simulink model "UPSControl"  (R2025b)
settings: Solver=VariableStepAuto  StartTime=0.0  StopTime=10  FixedStep=Ts  RelTol=1e-3
PostLoadFcn:
  | DataCenterParam;
values from neighbouring files (symbols this model uses):
  generator = struct    [GeneratorParam.m]
  lineInductance = 1e-6    (= 1e-06)    [DataCenterParam.m]    (also in GridParam.m)
  lineResistance = 1e-3    (= 0.001)    [DataCenterParam.m]    (also in GridParam.m)
  loadPower = 5e6    (= 5000000)    [DataCenterParam.m]    (also in LVRT.m; RedundancyAnalysis.m = 10000000)
  machine = struct    [GeneratorParam.m]
  powerTau = 0.005    [DataCenterParam.m]
  Ts = 5e-5    (= 5e-05)    [DataCenterParam.m]    (also in GeneratorParam.m)
  utilizationFactor = 0.45    [DataCenterParam.m]    (also in RedundancyAnalysis.m)
undefined symbols (not defined in the file or in its folder): breaker, ctLimitDelayTime, DiscIntNeverNeededParam, ee_sli_rtmsupport, gcbh, grid, rack, ups
libraries: nesl_utility x96, fl_lib x96, eeGeneralControl x84, ee_lib x80, simulink x68, eeTransforms x30, nesl_utility_internal x16, eeSinusoidalMeasurementV2 x13, slpidlib x12, simulink_extras x12, datacenter_lib x5, batteryecm_lib x4
(part 2 of 13)

== system UPSControl/ Back up Generator/Generator Set/Detailed ==
  PRef : Inport
  AVR and Exciter : Subsystem
  "Governor and Prime Mover " : Subsystem  mask(Governor and Prime Mover){pu_speed_reference=pu_speed_reference, droop_percentage=droop_percentage, pu_load_reference_setpoint=pu_load_reference_setpoint, T_G=T_G, T_CH=T_CH, base_torque=base_torque, pu_torque0=pu_torque0}
      mask prompts: pu_speed_reference "Speed reference, (pu)"; droop_percentage "Percentage droop, (%)"; pu_load_reference_setpoint "Load reference setpoint, (pu)"; T_G "Time constant of governor, (s)"; T_CH "Time constant of main inlet volumes and steam chest, (s)"; base_torque "Base torque, (N*m)"; pu_torque0 "Initial torque, (pu)"
      mask help:
      | Implements a synchronous machine governor and prime mover. The prime mover is a non-reheat steam turbine.
      |
      | The input to the block is a per-unit synchronous machine measurement vector.
      |
      | R and C are mechanical rotational ports.
  Inertia : ee_lib/Electromechanical/Mechanical/Machine Inertia  SRated=genRating*1000 V*A  FRated=frequency Hz  nPolePairs=polePairs  inertia_option=2  J=0.5754*200 kg*m^2  H=3.525*4 s*W/V/A  damper_option=2  D=39.0509 N*m/(rad/s)  pu_D=0.01  initialization_option=2  fMechanical0=30 Hz  fElectrical0=frequency Hz
      settings: InternalSimscapePortConfiguration="{\"Bottom\":[],\"Left\":[{\"id\":\"R\",\"label\":\"R\",\"type\":\"foundation.mechanical.rotational.rotational\"}],\"Right\":[],\"Top\":[]}"
  Machine : ee_lib/Electromechanical/Synchronous/Synchronous Machine Round Rotor  port_option=ee.enum.threePhasePort.composite  SRated=genRating*1000 A*V  VRated=Vac V  FRated=frequency Hz  nPolePairs=polePairs  param_option=ee.enum.sm.parameterization.standard  fieldCircuitParameterization_option=ee.enum.sm.fieldparameterization.voltage  baseEfd=200 V  baseIfd=1e-3%machine.fieldCurrent A  zero_sequence=ee.enum.park.zerosequence.exclude  axes_param=ee.enum.rotorangle.daxis  Ladu=1.66  Laqu=1.61  L0=0.15  Ll=0.05  Ra=machine.Ra  Lfd=0.165  Rfd=0.0006  L1d=0.1713  R1d=0.0284  L1q=0.7252  R1q=0.00619  L2q=0.125  R2q=0.02368  Xl=machine.Xl  Xd=machine.Xd  Xq=machine.Xq  X0=0.06  Xdd=machine.XdTransient  Xqd=machine.XqTransient  Xddd=machine.XdSubTransient  Xqdd=machine.XqSubTransient  d_option=ee.enum.circuit.open  Td0d=machine.tauDAxisTransient s  Tdd=0.03 s  Td0dd=machine.tauDAxisSubTransient s  Tddd=0.008 s  q_option=ee.enum.circuit.open  Tq0d=machine.tauQAxisTransient s  Tqd=0.03 s  Tq0dd=machine.tauQAxisSubTransient s  Tqdd=0.008 s  saturation_option=ee.enum.saturation.exclude  saturation_ifd=[0, .48, .76, 1.38, 1.79]  saturation_Vag=[0, .8, 1.08, 1.31, 1.4]  initialization_option=ee.enum.sm.initialization.electrical  source_type=ee.enum.sm.load_flow_source_type.Swing  Vmag0=machine.voltage V  Vang0=0 deg  Pt0=0 A*V  Qt0=0 A*V  minimum_pu=0.95  phase_search_range=[-inf, inf] deg  gmin=1e-6 S  connection_option=ee.enum.Connection.wye  num_q_dampers=2  rotor_offset=-pi / 2 rad  pu_psid_specify=off  pu_psid_priority=None  pu_psid=0  pu_psid_nominal_specify=off  pu_psid_nominal_value=1  pu_psid_nominal_unit=1  pu_psiq_specify=off  pu_psiq_priority=None  pu_psiq=0  pu_psiq_nominal_specify=off  pu_psiq_nominal_value=1  pu_psiq_nominal_unit=1  pu_psifd_specify=off  pu_psifd_priority=None  pu_psifd=0  pu_psifd_nominal_specify=off  pu_psifd_nominal_value=1  pu_psifd_nominal_unit=1  pu_psi1d_specify=off  pu_psi1d_priority=None  pu_psi1d=0  pu_psi1d_nominal_specify=off  pu_psi1d_nominal_value=1  pu_psi1d_nominal_unit=1  pu_psi1q_specify=off  pu_psi1q_priority=None  pu_psi1q=0  pu_psi1q_nominal_specify=off  pu_psi1q_nominal_value=1  pu_psi1q_nominal_unit=1  pu_psi2q_specify=off  pu_psi2q_priority=None  pu_psi2q=0  pu_psi2q_nominal_specify=off  pu_psi2q_nominal_value=1  pu_psi2q_nominal_unit=1  angular_position_diff_specify=off  angular_position_diff_priority=None  angular_position_diff=180 deg  angular_position_diff_nominal_specify=off  angular_position_diff_nominal_value=1  angular_position_diff_nominal_unit=deg  Tmeas=298.15 K  alpha=3.93e-3 1/K  stator_thermal_mass=100 J/K  rotor_thermal_mass=200 J/K  temperatureA_specify=off  temperatureA_priority=High  temperatureA=25 degC  temperatureA_nominal_specify=off  temperatureA_nominal_value=1  temperatureA_nominal_unit=degC  temperatureB_specify=off  temperatureB_priority=High  temperatureB=25 degC  temperatureB_nominal_specify=off  temperatureB_nominal_value=1  temperatureB_nominal_unit=degC  temperatureC_specify=off  temperatureC_priority=High  temperatureC=25 degC  temperatureC_nominal_specify=off  temperatureC_nominal_value=1  temperatureC_nominal_unit=degC  temperatureR_specify=off  temperatureR_priority=High  temperatureR=25 degC  temperatureR_nominal_specify=off  temperatureR_nominal_value=1  temperatureR_nominal_unit=degC
      settings: InternalSimscapePortConfiguration="{\"Bottom\":[],\"Left\":[{\"id\":\"fd_p\",\"label\":\"fd+\",\"type\":\"foundation.electrical.electrical\"},{\"id\":\"fd_n\",\"label\":\"fd-\",\"type\":\"foundation.electrical.electrical\"},{\"id\":\"R\",\"label\":\"R\",\"type\":\"foundation.mechanical.rotational.rotational\"},{\"id\":\"C\",\"label\":\"C\",\"type\":\"foundation.mechanical.rotational.rotational\"}],\"Right\":[{\"id\":\"pu_output\",\"label\":\"pu\",\"type\":\"output\"},{\"id\":\"N\",\"label\":\"~\",\"type\":\"foundation.electrical.three_phase\"}],\"Top\":[]}"
  Measurements : Subsystem
  ~ : PMIOPort  Side=Right
  Bus Element Out : Outport  PortName=Meas  Element=activePower
  BusElementOut : Outport  PortName=Meas  Element=reactivePower
  BusElementOut1 : Outport  PortName=Meas  Element=voltage
  BusElementOut2 : Outport  PortName=Meas  Element=current
  wires:
  Measurements/4(I) -> BusElementOut2/1
  Measurements/3(V) -> BusElementOut1/1
  Measurements/1(P) -> Bus Element Out/1
  Measurements/2(Q) -> BusElementOut/1
  PRef/1 -> "Governor and Prime Mover "/1(PRef)
  connections:
  ~/RConn1 -- Measurements/RConn1
  Measurements/LConn1 -- Machine/RConn2
  Machine/LConn1 -- AVR and Exciter/RConn1
  Machine/LConn4 -- "Governor and Prime Mover "/RConn2
  "Governor and Prime Mover "/RConn1 -- Machine/LConn3 -- Inertia/LConn1
  "Governor and Prime Mover "/LConn1 -- Machine/RConn1 -- AVR and Exciter/LConn1
  Machine/LConn2 -- AVR and Exciter/RConn2

== system UPSControl/ Back up Generator/Generator Set/Simplified ==
  PRef : Inport
  Electrical Reference : fl_lib/Electrical/Electrical Elements/Electrical Reference
  Exciter : Subsystem
  Machine : ee_lib/Electromechanical/Synchronous/Synchronous Machine Round Rotor  port_option=ee.enum.threePhasePort.composite  SRated=genRating kW  VRated=Vac V  FRated=frequency Hz  nPolePairs=polePairs  param_option=ee.enum.sm.parameterization.standard  fieldCircuitParameterization_option=ee.enum.sm.fieldparameterization.voltage  baseEfd=100 V  baseIfd=1300 A  zero_sequence=ee.enum.park.zerosequence.exclude  axes_param=ee.enum.rotorangle.daxis  Ladu=1.66  Laqu=1.61  L0=0.15  Ll=0.05  Ra=0.03/5  Lfd=0.165  Rfd=0.0006  L1d=0.1713  R1d=0.0284  L1q=0.7252  R1q=0.00619  L2q=0.125  R2q=0.02368  Xl=0.05/5  Xd=1.72/5  Xq=0.79/5  X0=0.06  Xdd=0.13/5  Xqd=0.17/3  Xddd=0.09/5  Xqdd=0.12/5  d_option=ee.enum.circuit.short  Td0d=0.75 s  Tdd=0.03 s  Td0dd=0.03 s  Tddd=0.008 s  q_option=ee.enum.circuit.open  Tq0d=0.6 s  Tqd=0.03 s  Tq0dd=0.02 s  Tqdd=0.008 s  saturation_option=ee.enum.saturation.exclude  saturation_ifd=[0, .48, .76, 1.38, 1.79]  saturation_Vag=[0, .8, 1.08, 1.31, 1.4]  initialization_option=ee.enum.sm.initialization.steadystate  source_type=ee.enum.sm.load_flow_source_type.Swing  Vmag0=6600 V  Vang0=0 deg  Pt0=0 A*V  Qt0=0 A*V  minimum_pu=0.95  phase_search_range=[-inf, inf] deg  gmin=1e-4 S  connection_option=ee.enum.Connection.wye  num_q_dampers=2  rotor_offset=-pi / 2 rad  pu_psid_specify=off  pu_psid_priority=None  pu_psid=0  pu_psid_nominal_specify=off  pu_psid_nominal_value=1  pu_psid_nominal_unit=1  pu_psiq_specify=off  pu_psiq_priority=None  pu_psiq=0  pu_psiq_nominal_specify=off  pu_psiq_nominal_value=1  pu_psiq_nominal_unit=1  pu_psifd_specify=off  pu_psifd_priority=None  pu_psifd=0  pu_psifd_nominal_specify=off  pu_psifd_nominal_value=1  pu_psifd_nominal_unit=1  pu_psi1d_specify=off  pu_psi1d_priority=None  pu_psi1d=0  pu_psi1d_nominal_specify=off  pu_psi1d_nominal_value=1  pu_psi1d_nominal_unit=1  pu_psi1q_specify=off  pu_psi1q_priority=None  pu_psi1q=0  pu_psi1q_nominal_specify=off  pu_psi1q_nominal_value=1  pu_psi1q_nominal_unit=1  pu_psi2q_specify=off  pu_psi2q_priority=None  pu_psi2q=0  pu_psi2q_nominal_specify=off  pu_psi2q_nominal_value=1  pu_psi2q_nominal_unit=1  angular_position_diff_specify=off  angular_position_diff_priority=None  angular_position_diff=180 deg  angular_position_diff_nominal_specify=off  angular_position_diff_nominal_value=1  angular_position_diff_nominal_unit=deg  Tmeas=298.15 K  alpha=3.93e-3 1/K  stator_thermal_mass=100 J/K  rotor_thermal_mass=200 J/K  temperatureA_specify=off  temperatureA_priority=High  temperatureA=25 degC  temperatureA_nominal_specify=off  temperatureA_nominal_value=1  temperatureA_nominal_unit=degC  temperatureB_specify=off  temperatureB_priority=High  temperatureB=25 degC  temperatureB_nominal_specify=off  temperatureB_nominal_value=1  temperatureB_nominal_unit=degC  temperatureC_specify=off  temperatureC_priority=High  temperatureC=25 degC  temperatureC_nominal_specify=off  temperatureC_nominal_value=1  temperatureC_nominal_unit=degC  temperatureR_specify=off  temperatureR_priority=High  temperatureR=25 degC  temperatureR_nominal_specify=off  temperatureR_nominal_value=1  temperatureR_nominal_unit=degC
      settings: InternalSimscapePortConfiguration="{\"Bottom\":[],\"Left\":[{\"id\":\"fd_p\",\"label\":\"fd+\",\"type\":\"foundation.electrical.electrical\"},{\"id\":\"fd_n\",\"label\":\"fd-\",\"type\":\"foundation.electrical.electrical\"},{\"id\":\"R\",\"label\":\"R\",\"type\":\"foundation.mechanical.rotational.rotational\"},{\"id\":\"C\",\"label\":\"C\",\"type\":\"foundation.mechanical.rotational.rotational\"}],\"Right\":[{\"id\":\"pu_output\",\"label\":\"pu\",\"type\":\"output\"},{\"id\":\"N\",\"label\":\"~\",\"type\":\"foundation.electrical.three_phase\"}],\"Top\":[]}"
  Machine Inertia : ee_lib/Electromechanical/Mechanical/Machine Inertia  SRated=genRating*1000 V*A  FRated=frequency Hz  nPolePairs=polePairs  inertia_option=1  J=0.5754 kg*m^2  H=3.525 s*W/V/A  damper_option=2  D=39.0509 N*m/(rad/s)  pu_D=0.01  initialization_option=2  fMechanical0=60 Hz  fElectrical0=60 Hz
      settings: InternalSimscapePortConfiguration="{\"Bottom\":[],\"Left\":[{\"id\":\"R\",\"label\":\"R\",\"type\":\"foundation.mechanical.rotational.rotational\"}],\"Right\":[],\"Top\":[]}"
  Measurements : Subsystem
  Prime Mover : Subsystem
  ~ : PMIOPort  Side=Right
  Bus Element Out : Outport  PortName=Meas  Element=activePower
  BusElementOut : Outport  PortName=Meas  Element=reactivePower
  BusElementOut1 : Outport  PortName=Meas  Element=voltage
  BusElementOut2 : Outport  PortName=Meas  Element=current
  wires:
  Measurements/2(Q) -> BusElementOut/1
  Measurements/1(P) -> Bus Element Out/1
  Measurements/3(V) -> BusElementOut1/1
  Measurements/4(I) -> BusElementOut2/1
  PRef/1 -> Prime Mover/1(PRef)
  connections:
  Measurements/LConn1 -- Machine/RConn2
  ~/RConn1 -- Measurements/RConn1
  Prime Mover/RConn2 -- Machine/LConn4
  Exciter/RConn1 -- Machine/LConn1
  Machine/LConn3 -- Prime Mover/RConn1 -- Machine Inertia/LConn1
  Electrical Reference/LConn1 -- Machine/LConn2 -- Exciter/RConn2

== system UPSControl/HV Substation/Transformer/Detailed ==
  Two-Winding Transformer (Three-Phase) : ee_lib/Passive/Transformers/Two-Winding Transformer (Three-Phase)  SRated=100e6 A*V  FRated=grid.frequency Hz  Winding1Connection=ee.enum.windingconnection.Yg  VRated1=grid.voltage V  Winding2Connection=ee.enum.windingconnection.Yg  VRated2=13200 V  CoreType=ee.enum.coretype.threelimb  pu_Rw1=0.01  pu_Rw2=0.01  leakage_reactance_option=ee.enum.transformer_leakage.include  pu_Xl1=0.05  pu_Xl2=0.05  magnetizing_resistance_option=ee.enum.transformer_magnetizingResistance.exclude  pu_Rm=500  magnetizing_reactance_option=ee.enum.transformer_magnetizingReactance.exclude  saturation_option=ee.enum.transformer_saturation.exclude  pu_Xm=500  current_data=[0, .002, 1, 2]  magnetic_flux_data=[0, 1.2, 1.5, 1.51]  pu_X0=0.5  i1_specify=off  i1_priority=None  i1=[0, 0, 0] A  i1_nominal_specify=off  i1_nominal_value=1  i1_nominal_unit=A  i2_specify=off  i2_priority=None  i2=[0, 0, 0] A  i2_nominal_specify=off  i2_nominal_value=1  i2_nominal_unit=A  phi_specify=off  phi_priority=None  phi=[0, 0, 0]  phi_nominal_specify=off  phi_nominal_value=1  phi_nominal_unit=1  power_dissipated_specify=off  power_dissipated_priority=None  power_dissipated=0 W  power_dissipated_nominal_specify=off  power_dissipated_nominal_value=1  power_dissipated_nominal_unit=W
      settings: InternalSimscapePortConfiguration="{\"Bottom\":[],\"Left\":[{\"id\":\"N1\",\"label\":\"~1\",\"type\":\"foundation.electrical.three_phase\"}],\"Right\":[{\"id\":\"N2\",\"label\":\"~2\",\"type\":\"foundation.electrical.three_phase\"}],\"Top\":[]}"
  In : PMIOPort  Side=Left
  Out : PMIOPort  Port=2  Side=Right
  connections:
  Two-Winding Transformer (Three-Phase)/LConn1 -- In/RConn1
  Two-Winding Transformer (Three-Phase)/RConn1 -- Out/RConn1

== system UPSControl/HV Substation/Transformer/Simplified ==
  Electrical Reference : fl_lib/Electrical/Electrical Elements/Electrical Reference
  Electrical Reference1 : fl_lib/Electrical/Electrical Elements/Electrical Reference
  Ideal Transformer : fl_lib/Electrical/Electrical Elements/Ideal Transformer  n=windingRatio  i1_specify=off  i1_priority=None  i1=0 A  i1_nominal_specify=off  i1_nominal_value=1  i1_nominal_unit=A  v1_specify=off  v1_priority=None  v1=0 V  v1_nominal_specify=off  v1_nominal_value=1  v1_nominal_unit=V  i2_specify=off  i2_priority=None  i2=0 A  i2_nominal_specify=off  i2_nominal_value=1  i2_nominal_unit=A  v2_specify=off  v2_priority=None  v2=0 V  v2_nominal_specify=off  v2_nominal_value=1  v2_nominal_unit=V
  Ideal Transformer1 : fl_lib/Electrical/Electrical Elements/Ideal Transformer  n=windingRatio  i1_specify=off  i1_priority=None  i1=0 A  i1_nominal_specify=off  i1_nominal_value=1  i1_nominal_unit=A  v1_specify=off  v1_priority=None  v1=0 V  v1_nominal_specify=off  v1_nominal_value=1  v1_nominal_unit=V  i2_specify=off  i2_priority=None  i2=0 A  i2_nominal_specify=off  i2_nominal_value=1  i2_nominal_unit=A  v2_specify=off  v2_priority=None  v2=0 V  v2_nominal_specify=off  v2_nominal_value=1  v2_nominal_unit=V
  Ideal Transformer2 : fl_lib/Electrical/Electrical Elements/Ideal Transformer  n=windingRatio  i1_specify=off  i1_priority=None  i1=0 A  i1_nominal_specify=off  i1_nominal_value=1  i1_nominal_unit=A  v1_specify=off  v1_priority=None  v1=0 V  v1_nominal_specify=off  v1_nominal_value=1  v1_nominal_unit=V  i2_specify=off  i2_priority=None  i2=0 A  i2_nominal_specify=off  i2_nominal_value=1  i2_nominal_unit=A  v2_specify=off  v2_priority=None  v2=0 V  v2_nominal_specify=off  v2_nominal_value=1  v2_nominal_unit=V
  Phase Splitter : ee_lib/Connectors & References/Phase Splitter
  Phase Splitter1 : ee_lib/Connectors & References/Phase Splitter
  In : PMIOPort  Side=Left
  Out : PMIOPort  Port=2  Side=Right
  connections:
  Ideal Transformer/RConn2 -- Electrical Reference1/LConn1 -- Ideal Transformer1/RConn2 -- Ideal Transformer2/RConn2
  Phase Splitter/RConn3 -- Ideal Transformer2/LConn1
  Phase Splitter/RConn2 -- Ideal Transformer1/LConn1
  Phase Splitter/RConn1 -- Ideal Transformer/LConn1
  Ideal Transformer/LConn2 -- Electrical Reference/LConn1 -- Ideal Transformer1/LConn2 -- Ideal Transformer2/LConn2
  Phase Splitter/LConn1 -- In/RConn1
  Phase Splitter1/LConn1 -- Out/RConn1
  Ideal Transformer/RConn1 -- Phase Splitter1/RConn1
  Ideal Transformer2/RConn1 -- Phase Splitter1/RConn3
  Ideal Transformer1/RConn1 -- Phase Splitter1/RConn2

== system UPSControl/MV Transformer/Transformer/Detailed ==
  Two-Winding Transformer (Three-Phase) : ee_lib/Passive/Transformers/Two-Winding Transformer (Three-Phase)  SRated=100e6 A*V  FRated=grid.frequency Hz  Winding1Connection=ee.enum.windingconnection.Yg  VRated1=13200 V  Winding2Connection=ee.enum.windingconnection.Yg  VRated2=ups.Vac V  CoreType=ee.enum.coretype.threelimb  pu_Rw1=0.01  pu_Rw2=0.01  leakage_reactance_option=ee.enum.transformer_leakage.include  pu_Xl1=0.05  pu_Xl2=0.05  magnetizing_resistance_option=ee.enum.transformer_magnetizingResistance.exclude  pu_Rm=500  magnetizing_reactance_option=ee.enum.transformer_magnetizingReactance.exclude  saturation_option=ee.enum.transformer_saturation.exclude  pu_Xm=500  current_data=[0, .002, 1, 2]  magnetic_flux_data=[0, 1.2, 1.5, 1.51]  pu_X0=0.5  i1_specify=off  i1_priority=None  i1=[0, 0, 0] A  i1_nominal_specify=off  i1_nominal_value=1  i1_nominal_unit=A  i2_specify=off  i2_priority=None  i2=[0, 0, 0] A  i2_nominal_specify=off  i2_nominal_value=1  i2_nominal_unit=A  phi_specify=off  phi_priority=None  phi=[0, 0, 0]  phi_nominal_specify=off  phi_nominal_value=1  phi_nominal_unit=1  power_dissipated_specify=off  power_dissipated_priority=None  power_dissipated=0 W  power_dissipated_nominal_specify=off  power_dissipated_nominal_value=1  power_dissipated_nominal_unit=W
      settings: InternalSimscapePortConfiguration="{\"Bottom\":[],\"Left\":[{\"id\":\"N1\",\"label\":\"~1\",\"type\":\"foundation.electrical.three_phase\"}],\"Right\":[{\"id\":\"N2\",\"label\":\"~2\",\"type\":\"foundation.electrical.three_phase\"}],\"Top\":[]}"
  In : PMIOPort  Side=Left
  Out : PMIOPort  Port=2  Side=Right
  connections:
  Two-Winding Transformer (Three-Phase)/LConn1 -- In/RConn1
  Two-Winding Transformer (Three-Phase)/RConn1 -- Out/RConn1

== system UPSControl/MV Transformer/Transformer/Simplified ==
  Electrical Reference : fl_lib/Electrical/Electrical Elements/Electrical Reference
  Electrical Reference1 : fl_lib/Electrical/Electrical Elements/Electrical Reference
  Ideal Transformer : fl_lib/Electrical/Electrical Elements/Ideal Transformer  n=windingRatio  i1_specify=off  i1_priority=None  i1=0 A  i1_nominal_specify=off  i1_nominal_value=1  i1_nominal_unit=A  v1_specify=off  v1_priority=None  v1=0 V  v1_nominal_specify=off  v1_nominal_value=1  v1_nominal_unit=V  i2_specify=off  i2_priority=None  i2=0 A  i2_nominal_specify=off  i2_nominal_value=1  i2_nominal_unit=A  v2_specify=off  v2_priority=None  v2=0 V  v2_nominal_specify=off  v2_nominal_value=1  v2_nominal_unit=V
  Ideal Transformer1 : fl_lib/Electrical/Electrical Elements/Ideal Transformer  n=windingRatio  i1_specify=off  i1_priority=None  i1=0 A  i1_nominal_specify=off  i1_nominal_value=1  i1_nominal_unit=A  v1_specify=off  v1_priority=None  v1=0 V  v1_nominal_specify=off  v1_nominal_value=1  v1_nominal_unit=V  i2_specify=off  i2_priority=None  i2=0 A  i2_nominal_specify=off  i2_nominal_value=1  i2_nominal_unit=A  v2_specify=off  v2_priority=None  v2=0 V  v2_nominal_specify=off  v2_nominal_value=1  v2_nominal_unit=V
  Ideal Transformer2 : fl_lib/Electrical/Electrical Elements/Ideal Transformer  n=windingRatio  i1_specify=off  i1_priority=None  i1=0 A  i1_nominal_specify=off  i1_nominal_value=1  i1_nominal_unit=A  v1_specify=off  v1_priority=None  v1=0 V  v1_nominal_specify=off  v1_nominal_value=1  v1_nominal_unit=V  i2_specify=off  i2_priority=None  i2=0 A  i2_nominal_specify=off  i2_nominal_value=1  i2_nominal_unit=A  v2_specify=off  v2_priority=None  v2=0 V  v2_nominal_specify=off  v2_nominal_value=1  v2_nominal_unit=V
  Phase Splitter : ee_lib/Connectors & References/Phase Splitter
  Phase Splitter1 : ee_lib/Connectors & References/Phase Splitter
  In : PMIOPort  Side=Left
  Out : PMIOPort  Port=2  Side=Right
  connections:
  Ideal Transformer/RConn2 -- Electrical Reference1/LConn1 -- Ideal Transformer1/RConn2 -- Ideal Transformer2/RConn2
  Phase Splitter/RConn3 -- Ideal Transformer2/LConn1
  Phase Splitter/RConn2 -- Ideal Transformer1/LConn1
  Phase Splitter/RConn1 -- Ideal Transformer/LConn1
  Ideal Transformer/LConn2 -- Electrical Reference/LConn1 -- Ideal Transformer1/LConn2 -- Ideal Transformer2/LConn2
  Phase Splitter/LConn1 -- In/RConn1
  Phase Splitter1/LConn1 -- Out/RConn1
  Ideal Transformer/RConn1 -- Phase Splitter1/RConn1
  Ideal Transformer2/RConn1 -- Phase Splitter1/RConn3
  Ideal Transformer1/RConn1 -- Phase Splitter1/RConn2

== system UPSControl/Server Load/Server Racks/PDU Racks ==
  PS Product : fl_lib/Physical Signals/Functions/PS Product
  Server Tray : Subsystem  mask{nGPU=nGPU, gpuTDPperDie=gpuTDPperDie, gpuIdlePower=gpuIdlePower, gpuHBMpower=gpuHBMpower, gpuExponent=gpuExponent, gpuHBMutil=gpuHBMutil, gpuLeakage=gpuLeakage, gpuNominalDieT=gpuNominalDieT, gpuDieThermalC=gpuDieThermalC, gpuHeatSinkR=gpuHeatSinkR, gpuSurfArea=gpuSurfArea, gpuAmbientR=gpuAmbientR, nCPU=nCPU, cpuTDPperSocket=cpuTDPperSocket, cpuIdlePower=cpuIdlePower, cpuExponent=cpuExponent, cpuLeakage=cpuLeakage, cpuNominalDieT=cpuNominalDieT, cpuDieThermalC=cpuDieThermalC, cpuHeatSinkR=cpuHeatSinkR, cpuSurfArea=cpuSurfArea, cpuAmbientR=cpuAmbientR, trayMass=trayMass, trayCp=trayCp, trayThermalR=trayThermalR, initialT=initialT, htc=htc}
      mask prompts: nGPU "Number of GPU (-)"; gpuTDPperDie "GPU TDP per die (W)"; gpuIdlePower "GPU idle power (W)"; gpuHBMpower "HBM power per GPU (W)"; gpuExponent "GPU power utilization exponent (-)"; gpuHBMutil "HBM utilization as fraction of compute utilization (-)"; gpuLeakage "Leakage increase per K above nominal temperature (W/K)"; gpuNominalDieT "Nominal die temperature at TDP (K)"; gpuDieThermalC "GPU die thermal capacitance (J/K)"; gpuHeatSinkR "GPU die-heat-sink thermal resistance (K/W)"; gpuSurfArea "Surface area per die for ambient heat transfer (m^2)"; gpuAmbientR "GPU die-ambient thermal resistance (K/W)"; nCPU "Number of CPU (-)"; cpuTDPperSocket "CPU TDP per socket (W)"; cpuIdlePower "CPU idle power per socket (W)"; cpuExponent "CPU power utilization exponent (-)"; cpuLeakage "Leakage increase per K above nominal temperature (W/K)"; cpuNominalDieT "Nominal die temperature at TDP (K)"; cpuDieThermalC "CPU die thermal capacitance (J/K)"; cpuHeatSinkR "CPU die-heat-sink thermal resistance (K/W)"; cpuSurfArea "Surface area per die for ambient heat transfer (m^2)"; cpuAmbientR "CPU die-ambient thermal resistance (K/W)"; trayMass "Tray mass (kg)"; trayCp "Tray specific heat capacity (J/kg*K)"; trayThermalR "Tray to external thermal resistance (K/W)"; initialT "Initial temperature (K)"; htc "Heat transfer coefficient to ambient (W/m^2.K)"
      settings: CopyFcn=set_param(gcbh,'LinkStatus','none');  PortSchema="{\"entries\":[{\"content\":{\"sides\":[{\"content\":{\"connectorIds\":[\"LConn1\",\"LConn2\",\"LConn3\"]},\"type\":\"ConnectorPlacement.EquallySpacedRectSide\",\"uuid\":\"893f21b9-92d6-433a-96e5-f8193a696c29\"},{\"content\":{\"connectorIds\":[\"RConn1\",\"RConn2\",\"RConn3\"],\"side\":\"RIGHT\"},\"type\":\"ConnectorPlacement.EquallySpacedRectSide\",\"uuid\":\"efd10409-70d8-4a6a-97a2-13f0e6f538e3\"},{\"content\":{\"side\":\"TOP\"},\"type\":\"ConnectorPlacement.EquallySpacedRectSide\",\"uuid\":\"8c9765cd-90e6-46de-916c-606bbb93143e\"},{\"content\":{\"connectorIds\":[\"RConn4\"],\"side\":\"BOTTOM\"},\"type\":\"ConnectorPlacement.EquallySpacedRectSide\",\"uuid\":\"9656b44e-d582-43b0-a7fe-c629821d6c27\"}]},\"type\":\"ConnectorPlacement.EquallySpacedConnector\",\"uuid\":\"add7a682-eb4b-4f46-a5b9-e161ccf96de5\"}],\"packageUris\":[\"http://schema.mathworks.com/mf0/Connector/R2020b\"],\"version\":\"1.0\"}"
      mask Help: web("DocumentationServerTray.html")
      mask DialogControl Container6 Prompt: GPU
      mask DialogControl Container7 Prompt: CPU
      mask DialogControl Container9 Prompt: IT Tray
      mask DialogControl Container8 Prompt: Initial Conditions
      mask Display: image('icon_serverPlate.png');
  TMamb : datacenter_lib/Thermal Multiplier
      settings: InternalSimscapePortConfiguration="{\"Bottom\":[],\"Left\":[{\"id\":\"A\",\"label\":\"A\",\"type\":\"foundation.thermal.thermal\"}],\"Right\":[{\"id\":\"B\",\"label\":\"B\",\"type\":\"foundation.thermal.thermal\"}],\"Top\":[{\"id\":\"Na\",\"label\":\"Na\",\"type\":\"input\"},{\"id\":\"Nb\",\"label\":\"Nb\",\"type\":\"input\"}]}"
  TMcdu : datacenter_lib/Thermal Multiplier
      settings: InternalSimscapePortConfiguration="{\"Bottom\":[],\"Left\":[{\"id\":\"A\",\"label\":\"A\",\"type\":\"foundation.thermal.thermal\"}],\"Right\":[{\"id\":\"B\",\"label\":\"B\",\"type\":\"foundation.thermal.thermal\"}],\"Top\":[{\"id\":\"Na\",\"label\":\"Na\",\"type\":\"input\"},{\"id\":\"Nb\",\"label\":\"Nb\",\"type\":\"input\"}]}"
  nTraysXnRacks : fl_lib/Physical Signals/Sources/PS Constant  constant=nTrays*nRacks
  one : fl_lib/Physical Signals/Sources/PS Constant  constant=1
  U_gpu : PMIOPort  Side=Left
  U_cpu : PMIOPort  Port=2  Side=Left
  Ha : PMIOPort  Port=3  Side=Left
  P : PMIOPort  Port=4  Side=Right
  T_gpu : PMIOPort  Port=5  Side=Right
  T_cpu : PMIOPort  Port=6  Side=Right
  Hc : PMIOPort  Port=7  Side=Right
  connections:
  Server Tray/LConn1 -- U_gpu/RConn1
  TMamb/LConn1 -- Ha/RConn1
  Server Tray/RConn2 -- T_gpu/RConn1
  TMcdu/RConn1 -- Hc/RConn1
  Server Tray/LConn2 -- U_cpu/RConn1
  Server Tray/RConn3 -- T_cpu/RConn1
  one/RConn1 -- TMcdu/LConn3 -- TMamb/LConn2
  Server Tray/RConn4 -- TMcdu/LConn1
  Server Tray/LConn3 -- TMamb/RConn1
  nTraysXnRacks/RConn1 -- PS Product/LConn1 -- TMcdu/LConn2 -- TMamb/LConn3
  Server Tray/RConn1 -- PS Product/LConn2
  PS Product/RConn1 -- P/RConn1

== system UPSControl/Server Load/UPS Units/Single UPS ==
  iChrg : Inport
  Bus Selector2 : BusSelector  OutputSignals=activePower,reactivePower
  Gain : Gain  Gain=5
  Gain1 : Gain  Gain=5
  RLC (Three-Phase)1 : ee_lib/Passive/RLC Assemblies/RLC (Three-Phase)  port_option=ee.enum.threePhasePort.composite  component_structure=ee.enum.rlc.structure.SeriesRL  R=1e-3 Ohm  L=1e-5 H  C=1e-6 F  R_parasitic=0 Ohm  G_parasitic=0 1/Ohm  IL_specify=on  IL_priority=None  IL=[0, 0, 0] A  IL_nominal_specify=off  IL_nominal_value=1  IL_nominal_unit=A  VC_specify=off  VC_priority=High  VC=[0, 0, 0] V  VC_nominal_specify=off  VC_nominal_value=1  VC_nominal_unit=V
      settings: InternalSimscapePortConfiguration="{\"Bottom\":[],\"Left\":[{\"id\":\"N1\",\"label\":\"~1\",\"type\":\"foundation.electrical.three_phase\"}],\"Right\":[{\"id\":\"N2\",\"label\":\"~2\",\"type\":\"foundation.electrical.three_phase\"}],\"Top\":[]}"
  UPS : Subsystem  VariantControl=Detailed  mask(Double-conversion Uniterrupted Power Supply (UPS)){plantRating=ups.rating, Vac=ups.Vac, frequency=ups.frequency, baseVoltageDC=ups.Vdc, sampleTime=ups.sampleTime, filterInductanceAFE=ups.AFE.filterInductance, filterResistanceAFE=ups.AFE.filterResistance/10, capacitance=ups.DCBus.capacitance, vBattNom=ups.batt.Vnom, iBatt=ups.batt.iRated, vBattMax=ups.batt.VMax, droopGain=ups.DCBus.droop, rampRate=ups.batt.rampRate, vGridMin=ups.DCBus.gridThreshold, vDCThreshold=ups.DCBus.VThreshold, initialMode=ups.batt.initialMode, kpDC=500%ups.DCBus.kpConverter/10, kiDC=500%ups.DCBus.kiConverter/10, bessConverterEfficiency=ups.DCBus.converterEff, filterInductance=ups.inverter.filterInductance, filterResistance=ups.inverter.filterResistance}
      mask prompts: plantRating "UPS Rating (kW)"; Vac "Rated AC side voltage (phase-phase RMS) (V)"; frequency "Rated electrical frequency at AC side (Hz)"; baseVoltageDC "Voltage on DC side (V)"; sampleTime "Sample time (s)"; filterInductanceAFE "Filter inductance (H)"; filterResistanceAFE "Filter resistance (Ohm)"; capacitance "Capacitance (F)"; vBattNom "Battery nominal voltage (V)"; iBatt "Battery rated current (A)"; vBattMax "Maximum battery voltage (V)"; droopGain "DC bus droop gain"; rampRate "Ramp rate for battery discharge"; vGridMin "Minimum grid voltage (V)"; vDCThreshold "Threshold DC Bus voltage (V)"; initialMode "Initial operating mode"; kpDC "DC-DC Converter proportional gain"; kiDC "DC-DC Converter integral gain"; bessConverterEfficiency "DC-DC converter efficiency (%)"; filterInductance "Filter inductance (H)"; filterResistance "Filter series resistance (Ohm)"
      mask help: This block models a double conversion uninterruptible power supply that continuously supplies the load through an inverter. It isolates the load from input disturbances and uses a battery on the DC link to maintain uninterrupted power during input outages.
      mask Help: web('UPS.html')
      mask DialogControl generalDetailed Prompt: General
      mask DialogControl Container9 Prompt: Active Front End
      mask DialogControl editRectifier Prompt: Edit converter parameters
      mask DialogControl editRectifier Callback:
      | blockPath = [gcb,'/','Rectifier','/','AC-DC Converter'];
      |     component.mask.openBlock(blockPath);
      mask DialogControl configureAFEController Prompt: Edit AFE controller
      mask DialogControl configureAFEController Callback:
      | blockPath = [gcb,'/','Rectifier','/','PFC Rectifier Controller'];
      |     component.mask.openBlock(blockPath);
      mask DialogControl cellDetailed Prompt: DC Link
      mask DialogControl configureBattery Prompt: Edit battery parameters
      mask DialogControl configureBattery Callback:
      | blockPath = [gcb,'/','DC-Link','/','BESS','/','Battery'] ;
      |     component.mask.openBlock(blockPath);
      mask DialogControl controllerDetailed Prompt: Inverter
      mask DialogControl editInverter Prompt: Edit converter parameters
      mask DialogControl editInverter Callback:
      | blockPath = [gcb,'/','Inverter','/','DC- AC Converter'];
      |     component.mask.openBlock(blockPath);
      mask DialogControl editInverterController Prompt: Edit inverter controller
      mask DialogControl editInverterController Callback:
      | blockPath = [gcb,'/','Inverter','/','Inverter Controller'] ;
      |     component.mask.openBlock(blockPath);
  GridSide : PMIOPort  Side=Left
  LoadSide : PMIOPort  Port=2  Side=Right
  Meas : Outport
  P : Outport  Port=2
  Q : Outport  Port=3
  wires:
  iChrg/1 -> UPS/1(iChrg)
  UPS/1(Meas) -> Bus Selector2/1, Meas/1
  Bus Selector2/2 -> Gain1/1  "<reactivePower>"
  Bus Selector2/1 -> Gain/1  "<activePower>"
  Gain/1 -> P/1
  Gain1/1 -> Q/1
  connections:
  GridSide/RConn1 -- UPS/LConn1
  RLC (Three-Phase)1/RConn1 -- LoadSide/RConn1
  UPS/RConn1 -- RLC (Three-Phase)1/LConn1

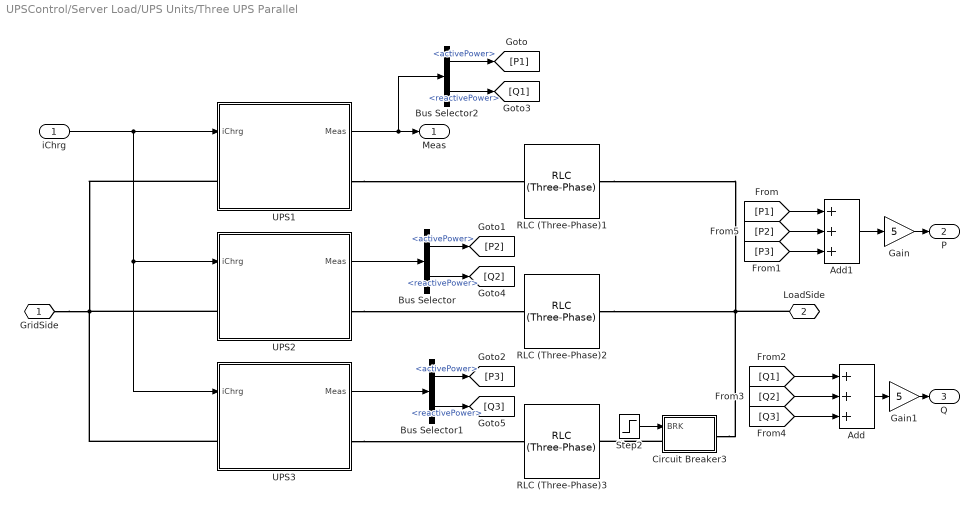
== system UPSControl/Server Load/UPS Units/Three UPS Parallel ==
  iChrg : Inport
  Add : Sum  Inputs=+++
  Add1 : Sum  Inputs=+++
  Bus Selector : BusSelector  OutputSignals=activePower,reactivePower
  Bus Selector1 : BusSelector  OutputSignals=activePower,reactivePower
  Bus Selector2 : BusSelector  OutputSignals=activePower,reactivePower
  Circuit Breaker3 : Subsystem
  Gain : Gain  Gain=5
  Gain1 : Gain  Gain=5
  RLC (Three-Phase)1 : ee_lib/Passive/RLC Assemblies/RLC (Three-Phase)  port_option=ee.enum.threePhasePort.composite  component_structure=ee.enum.rlc.structure.SeriesRL  R=1e-3 Ohm  L=1e-5 H  C=1e-6 F  R_parasitic=0 Ohm  G_parasitic=0 1/Ohm  IL_specify=on  IL_priority=None  IL=[0, 0, 0] A  IL_nominal_specify=off  IL_nominal_value=1  IL_nominal_unit=A  VC_specify=off  VC_priority=High  VC=[0, 0, 0] V  VC_nominal_specify=off  VC_nominal_value=1  VC_nominal_unit=V
      settings: InternalSimscapePortConfiguration="{\"Bottom\":[],\"Left\":[{\"id\":\"N1\",\"label\":\"~1\",\"type\":\"foundation.electrical.three_phase\"}],\"Right\":[{\"id\":\"N2\",\"label\":\"~2\",\"type\":\"foundation.electrical.three_phase\"}],\"Top\":[]}"
  RLC (Three-Phase)2 : ee_lib/Passive/RLC Assemblies/RLC (Three-Phase)  port_option=ee.enum.threePhasePort.composite  component_structure=ee.enum.rlc.structure.SeriesRL  R=1e-3 Ohm  L=1e-5 H  C=1e-6 F  R_parasitic=0 Ohm  G_parasitic=0 1/Ohm  IL_specify=on  IL_priority=None  IL=[0, 0, 0] A  IL_nominal_specify=off  IL_nominal_value=1  IL_nominal_unit=A  VC_specify=off  VC_priority=High  VC=[0, 0, 0] V  VC_nominal_specify=off  VC_nominal_value=1  VC_nominal_unit=V
      settings: InternalSimscapePortConfiguration="{\"Bottom\":[],\"Left\":[{\"id\":\"N1\",\"label\":\"~1\",\"type\":\"foundation.electrical.three_phase\"}],\"Right\":[{\"id\":\"N2\",\"label\":\"~2\",\"type\":\"foundation.electrical.three_phase\"}],\"Top\":[]}"
  RLC (Three-Phase)3 : ee_lib/Passive/RLC Assemblies/RLC (Three-Phase)  port_option=ee.enum.threePhasePort.composite  component_structure=ee.enum.rlc.structure.SeriesRL  R=1e-3 Ohm  L=1e-5 H  C=1e-6 F  R_parasitic=0 Ohm  G_parasitic=0 1/Ohm  IL_specify=on  IL_priority=None  IL=[0, 0, 0] A  IL_nominal_specify=off  IL_nominal_value=1  IL_nominal_unit=A  VC_specify=off  VC_priority=High  VC=[0, 0, 0] V  VC_nominal_specify=off  VC_nominal_value=1  VC_nominal_unit=V
      settings: InternalSimscapePortConfiguration="{\"Bottom\":[],\"Left\":[{\"id\":\"N1\",\"label\":\"~1\",\"type\":\"foundation.electrical.three_phase\"}],\"Right\":[{\"id\":\"N2\",\"label\":\"~2\",\"type\":\"foundation.electrical.three_phase\"}],\"Top\":[]}"
  Step2 : Step  Time=breaker.UPS  SampleTime=0
  UPS1 : Subsystem  VariantControl=Detailed  mask(Double-conversion Uniterrupted Power Supply (UPS)){plantRating=ups.rating, Vac=ups.Vac, frequency=ups.frequency, baseVoltageDC=ups.Vdc, sampleTime=ups.sampleTime, filterInductanceAFE=ups.AFE.filterInductance, filterResistanceAFE=ups.AFE.filterResistance, capacitance=ups.DCBus.capacitance, vBattNom=ups.batt.Vnom, iBatt=ups.batt.iRated, vBattMax=ups.batt.VMax, droopGain=ups.DCBus.droop, rampRate=ups.batt.rampRate, vGridMin=ups.DCBus.gridThreshold, vDCThreshold=ups.DCBus.VThreshold, initialMode=ups.batt.initialMode, kpDC=ups.DCBus.kpConverter, kiDC=ups.DCBus.kiConverter, bessConverterEfficiency=ups.DCBus.converterEff, filterInductance=ups.inverter.filterInductance, filterResistance=ups.inverter.filterResistance}
      mask prompts: plantRating "UPS Rating (kW)"; Vac "Rated AC side voltage (phase-phase RMS) (V)"; frequency "Rated electrical frequency at AC side (Hz)"; baseVoltageDC "Voltage on DC side (V)"; sampleTime "Sample time (s)"; filterInductanceAFE "Filter inductance (H)"; filterResistanceAFE "Filter resistance (Ohm)"; capacitance "Capacitance (F)"; vBattNom "Battery nominal voltage (V)"; iBatt "Battery rated current (A)"; vBattMax "Maximum battery voltage (V)"; droopGain "DC bus droop gain"; rampRate "Ramp rate for battery discharge"; vGridMin "Minimum grid voltage (V)"; vDCThreshold "Threshold DC Bus voltage (V)"; initialMode "Initial operating mode"; kpDC "DC-DC Converter proportional gain"; kiDC "DC-DC Converter integral gain"; bessConverterEfficiency "DC-DC converter efficiency (%)"; filterInductance "Filter inductance (H)"; filterResistance "Filter series resistance (Ohm)"
      mask help: This block models a double conversion uninterruptible power supply that continuously supplies the load through an inverter. It isolates the load from input disturbances and uses a battery on the DC link to maintain uninterrupted power during input outages.
      mask Help: web('UPS.html')
      mask DialogControl generalDetailed Prompt: General
      mask DialogControl Container9 Prompt: Active Front End
      mask DialogControl editRectifier Prompt: Edit converter parameters
      mask DialogControl editRectifier Callback:
      | blockPath = [gcb,'/','Rectifier','/','AC-DC Converter'];
      |     component.mask.openBlock(blockPath);
      mask DialogControl configureAFEController Prompt: Edit AFE controller
      mask DialogControl configureAFEController Callback:
      | blockPath = [gcb,'/','Rectifier','/','PFC Rectifier Controller'];
      |     component.mask.openBlock(blockPath);
      mask DialogControl cellDetailed Prompt: DC Link
      mask DialogControl configureBattery Prompt: Edit battery parameters
      mask DialogControl configureBattery Callback:
      | blockPath = [gcb,'/','DC-Link','/','BESS','/','Battery'] ;
      |     component.mask.openBlock(blockPath);
      mask DialogControl controllerDetailed Prompt: Inverter
      mask DialogControl editInverter Prompt: Edit converter parameters
      mask DialogControl editInverter Callback:
      | blockPath = [gcb,'/','Inverter','/','DC- AC Converter'];
      |     component.mask.openBlock(blockPath);
      mask DialogControl editInverterController Prompt: Edit inverter controller
      mask DialogControl editInverterController Callback:
      | blockPath = [gcb,'/','Inverter','/','Inverter Controller'] ;
      |     component.mask.openBlock(blockPath);
  UPS2 : Subsystem  VariantControl=Detailed  mask(Double-conversion Uniterrupted Power Supply (UPS)){plantRating=ups.rating, Vac=ups.Vac, frequency=ups.frequency, baseVoltageDC=ups.Vdc, sampleTime=ups.sampleTime, filterInductanceAFE=ups.AFE.filterInductance, filterResistanceAFE=ups.AFE.filterResistance, capacitance=ups.DCBus.capacitance, vBattNom=ups.batt.Vnom, iBatt=ups.batt.iRated, vBattMax=ups.batt.VMax, droopGain=ups.DCBus.droop, rampRate=ups.batt.rampRate, vGridMin=ups.DCBus.gridThreshold, vDCThreshold=ups.DCBus.VThreshold, initialMode=ups.batt.initialMode, kpDC=ups.DCBus.kpConverter, kiDC=ups.DCBus.kiConverter, bessConverterEfficiency=ups.DCBus.converterEff, filterInductance=ups.inverter.filterInductance, filterResistance=ups.inverter.filterResistance}
      mask prompts: plantRating "UPS Rating (kW)"; Vac "Rated AC side voltage (phase-phase RMS) (V)"; frequency "Rated electrical frequency at AC side (Hz)"; baseVoltageDC "Voltage on DC side (V)"; sampleTime "Sample time (s)"; filterInductanceAFE "Filter inductance (H)"; filterResistanceAFE "Filter resistance (Ohm)"; capacitance "Capacitance (F)"; vBattNom "Battery nominal voltage (V)"; iBatt "Battery rated current (A)"; vBattMax "Maximum battery voltage (V)"; droopGain "DC bus droop gain"; rampRate "Ramp rate for battery discharge"; vGridMin "Minimum grid voltage (V)"; vDCThreshold "Threshold DC Bus voltage (V)"; initialMode "Initial operating mode"; kpDC "DC-DC Converter proportional gain"; kiDC "DC-DC Converter integral gain"; bessConverterEfficiency "DC-DC converter efficiency (%)"; filterInductance "Filter inductance (H)"; filterResistance "Filter series resistance (Ohm)"
      mask help: This block models a double conversion uninterruptible power supply that continuously supplies the load through an inverter. It isolates the load from input disturbances and uses a battery on the DC link to maintain uninterrupted power during input outages.
      mask Help: web('UPS.html')
      mask DialogControl generalDetailed Prompt: General
      mask DialogControl Container9 Prompt: Active Front End
      mask DialogControl editRectifier Prompt: Edit converter parameters
      mask DialogControl editRectifier Callback:
      | blockPath = [gcb,'/','Rectifier','/','AC-DC Converter'];
      |     component.mask.openBlock(blockPath);
      mask DialogControl configureAFEController Prompt: Edit AFE controller
      mask DialogControl configureAFEController Callback:
      | blockPath = [gcb,'/','Rectifier','/','PFC Rectifier Controller'];
      |     component.mask.openBlock(blockPath);
      mask DialogControl cellDetailed Prompt: DC Link
      mask DialogControl configureBattery Prompt: Edit battery parameters
      mask DialogControl configureBattery Callback:
      | blockPath = [gcb,'/','DC-Link','/','BESS','/','Battery'] ;
      |     component.mask.openBlock(blockPath);
      mask DialogControl controllerDetailed Prompt: Inverter
      mask DialogControl editInverter Prompt: Edit converter parameters
      mask DialogControl editInverter Callback:
      | blockPath = [gcb,'/','Inverter','/','DC- AC Converter'];
      |     component.mask.openBlock(blockPath);
      mask DialogControl editInverterController Prompt: Edit inverter controller
      mask DialogControl editInverterController Callback:
      | blockPath = [gcb,'/','Inverter','/','Inverter Controller'] ;
      |     component.mask.openBlock(blockPath);
  UPS3 : Subsystem  VariantControl=Detailed  mask(Double-conversion Uniterrupted Power Supply (UPS)){plantRating=ups.rating, Vac=ups.Vac, frequency=ups.frequency, baseVoltageDC=ups.Vdc, sampleTime=ups.sampleTime, filterInductanceAFE=ups.AFE.filterInductance, filterResistanceAFE=ups.AFE.filterResistance, capacitance=ups.DCBus.capacitance, vBattNom=ups.batt.Vnom, iBatt=ups.batt.iRated, vBattMax=ups.batt.VMax, droopGain=ups.DCBus.droop, rampRate=ups.batt.rampRate, vGridMin=ups.DCBus.gridThreshold, vDCThreshold=ups.DCBus.VThreshold, initialMode=ups.batt.initialMode, kpDC=ups.DCBus.kpConverter, kiDC=ups.DCBus.kiConverter, bessConverterEfficiency=ups.DCBus.converterEff, filterInductance=ups.inverter.filterInductance, filterResistance=ups.inverter.filterResistance}
      mask prompts: plantRating "UPS Rating (kW)"; Vac "Rated AC side voltage (phase-phase RMS) (V)"; frequency "Rated electrical frequency at AC side (Hz)"; baseVoltageDC "Voltage on DC side (V)"; sampleTime "Sample time (s)"; filterInductanceAFE "Filter inductance (H)"; filterResistanceAFE "Filter resistance (Ohm)"; capacitance "Capacitance (F)"; vBattNom "Battery nominal voltage (V)"; iBatt "Battery rated current (A)"; vBattMax "Maximum battery voltage (V)"; droopGain "DC bus droop gain"; rampRate "Ramp rate for battery discharge"; vGridMin "Minimum grid voltage (V)"; vDCThreshold "Threshold DC Bus voltage (V)"; initialMode "Initial operating mode"; kpDC "DC-DC Converter proportional gain"; kiDC "DC-DC Converter integral gain"; bessConverterEfficiency "DC-DC converter efficiency (%)"; filterInductance "Filter inductance (H)"; filterResistance "Filter series resistance (Ohm)"
      mask help: This block models a double conversion uninterruptible power supply that continuously supplies the load through an inverter. It isolates the load from input disturbances and uses a battery on the DC link to maintain uninterrupted power during input outages.
      mask Help: web('UPS.html')
      mask DialogControl generalDetailed Prompt: General
      mask DialogControl Container9 Prompt: Active Front End
      mask DialogControl editRectifier Prompt: Edit converter parameters
      mask DialogControl editRectifier Callback:
      | blockPath = [gcb,'/','Rectifier','/','AC-DC Converter'];
      |     component.mask.openBlock(blockPath);
      mask DialogControl configureAFEController Prompt: Edit AFE controller
      mask DialogControl configureAFEController Callback:
      | blockPath = [gcb,'/','Rectifier','/','PFC Rectifier Controller'];
      |     component.mask.openBlock(blockPath);
      mask DialogControl cellDetailed Prompt: DC Link
      mask DialogControl configureBattery Prompt: Edit battery parameters
      mask DialogControl configureBattery Callback:
      | blockPath = [gcb,'/','DC-Link','/','BESS','/','Battery'] ;
      |     component.mask.openBlock(blockPath);
      mask DialogControl controllerDetailed Prompt: Inverter
      mask DialogControl editInverter Prompt: Edit converter parameters
      mask DialogControl editInverter Callback:
      | blockPath = [gcb,'/','Inverter','/','DC- AC Converter'];
      |     component.mask.openBlock(blockPath);
      mask DialogControl editInverterController Prompt: Edit inverter controller
      mask DialogControl editInverterController Callback:
      | blockPath = [gcb,'/','Inverter','/','Inverter Controller'] ;
      |     component.mask.openBlock(blockPath);
  GridSide : PMIOPort  Side=Left
  LoadSide : PMIOPort  Port=2  Side=Right
  Meas : Outport
  P : Outport  Port=2
  Q : Outport  Port=3
  wires:
  iChrg/1 -> UPS3/1(iChrg), UPS2/1(iChrg), UPS1/1(iChrg)
  UPS1/1(Meas) -> Bus Selector2/1, Meas/1
  UPS2/1(Meas) -> Bus Selector/1
  UPS3/1(Meas) -> Bus Selector1/1
  Bus Selector2/1 -> [P1]  "<activePower>"
  Bus Selector2/2 -> [Q1]  "<reactivePower>"
  Bus Selector/1 -> [P2]  "<activePower>"
  Bus Selector/2 -> [Q2]  "<reactivePower>"
  Bus Selector1/1 -> [P3]  "<activePower>"
  Bus Selector1/2 -> [Q3]  "<reactivePower>"
  [Q1] -> Add/1
  [Q2] -> Add/2
  [Q3] -> Add/3
  [P3] -> Add1/3
  [P2] -> Add1/2
  [P1] -> Add1/1
  Add1/1 -> Gain/1
  Gain/1 -> P/1
  Add/1 -> Gain1/1
  Gain1/1 -> Q/1
  Step2/1 -> Circuit Breaker3/1(BRK)
  connections:
  GridSide/RConn1 -- UPS3/LConn1 -- UPS2/LConn1 -- UPS1/LConn1
  UPS2/RConn1 -- RLC (Three-Phase)2/LConn1
  UPS3/RConn1 -- RLC (Three-Phase)3/LConn1
  UPS1/RConn1 -- RLC (Three-Phase)1/LConn1
  LoadSide/RConn1 -- RLC (Three-Phase)1/RConn1 -- RLC (Three-Phase)2/RConn1 -- Circuit Breaker3/RConn1
  Circuit Breaker3/LConn1 -- RLC (Three-Phase)3/RConn1

== system UPSControl/ Back up Generator/Generator Set/Detailed/AVR and Exciter ==
  AVR : eeSmDC2C/SM DC2C  E_FD0=1.01  Ts=Ts  R_C=0  X_C=0  T_R=0  K_A=300  T_A=0.06  T_B=0  T_C=0  K_F=0.058  T_F=0.62  V_Rmax=4.5  V_Rmin=-4.5  oelInputLocation=Unused  uelInputLocation=Unused  sclInputLocation=Unused  K_E=1  T_E=1.33  E_FDmin=-99  E_1=3.05  S_E_E1=0.279  E_2=2.29  S_E_E2=0.117
  Constant{3,5..9} (6 alike) : Constant  Value=0
  Constant4 : Constant  Value=1.05
  "E_FD Simulink-PS " : nesl_utility/Simulink-PS Converter  PhysicalDomain=network_engine_domain  SubClassName=ps_input  LeftPortType=input  RightPortType=output  PseudoPeriodic=off  Frequencies=[]  NoiseDistribution=none  NoiseParameters=[]  Unit=1  AffineConversion=off  FilteringAndDerivatives=provide  SimscapeFilterOrder=1  InputFilterTimeConstant=.001  UdotUserProvided=0
  Exciter : ee_lib/Electromechanical/Synchronous/Synchronous Machine Field Circuit  unit_option=ee.enum.unit.pu  SRated=machine.ratedPower*1000 V*A  FRated=machine.frequency Hz  fieldCircuitParameterization_option=ee.enum.sm.fieldparameterization.voltage  baseEfd=200 V  baseIfd=1e-3%machine.fieldCurrent A  parameterization_option=2  Ladu=1.66  Rfd=0.0006  Xl=machine.Xl  Xd=machine.Xd  Xdd=machine.XdTransient  Xddd=machine.XdSubTransient  d_option=ee.enum.circuit.open  Td0d=machine.tauDAxisTransient s  Tdd=0.03 s  Td0dd=machine.tauDAxisSubTransient s  Tddd=0.008 s
      settings: InternalSimscapePortConfiguration="{\"Bottom\":[],\"Left\":[{\"id\":\"Efd_pu\",\"label\":\"Efd_pu\",\"type\":\"input\"},{\"id\":\"Ifd_pu\",\"label\":\"Ifd_pu\",\"type\":\"output\"}],\"Right\":[{\"id\":\"fd_p\",\"label\":\"fd+\",\"type\":\"foundation.electrical.electrical\"},{\"id\":\"fd_n\",\"label\":\"fd-\",\"type\":\"foundation.electrical.electrical\"}],\"Top\":[]}"
  I_FD PS-Simulink : nesl_utility/PS-Simulink Converter  PhysicalDomain=network_engine_domain  SubClassName=ps_output  LeftPortType=input  RightPortType=output  PseudoPeriodic=off  Frequencies=[]  VectorFormat=1-D array  Unit=1  AffineConversion=off
  Terminal Current Measurement : ee_lib/Electromechanical/Synchronous/Synchronous Machine Measurement  output_idx=15
      settings: InternalSimscapePortConfiguration="{\"Bottom\":[],\"Left\":[{\"id\":\"pu_input\",\"label\":\"pu\",\"type\":\"input\"}],\"Right\":[{\"id\":\"pu_output\",\"label\":\"o\",\"type\":\"output\"}],\"Top\":[]}"
  Terminal Current PS-Simulink : nesl_utility/PS-Simulink Converter  PhysicalDomain=network_engine_domain  SubClassName=ps_output  LeftPortType=input  RightPortType=output  PseudoPeriodic=off  Frequencies=[]  VectorFormat=1-D array  Unit=1  AffineConversion=off
  Terminal Voltage Measurement : ee_lib/Electromechanical/Synchronous/Synchronous Machine Measurement  output_idx=14
      settings: InternalSimscapePortConfiguration="{\"Bottom\":[],\"Left\":[{\"id\":\"pu_input\",\"label\":\"pu\",\"type\":\"input\"}],\"Right\":[{\"id\":\"pu_output\",\"label\":\"o\",\"type\":\"output\"}],\"Top\":[]}"
  Terminal Voltage PS-Simulink : nesl_utility/PS-Simulink Converter  PhysicalDomain=network_engine_domain  SubClassName=ps_output  LeftPortType=input  RightPortType=output  PseudoPeriodic=off  Frequencies=[]  VectorFormat=1-D array  Unit=1  AffineConversion=off
  Terminator : Terminator
  Unit Delay : UnitDelay  InitialCondition=1.32943  SampleTime=-1
  pu : PMIOPort  Side=Left
  fd+ : PMIOPort  Port=2  Side=Right
  fd- : PMIOPort  Port=3  Side=Right
  wires:
  Unit Delay/1 -> Terminator/1
  I_FD PS-Simulink/1 -> Unit Delay/1
  Terminal Voltage PS-Simulink/1 -> AVR/3
  Constant3/1 -> AVR/2
  Constant4/1 -> AVR/1
  Constant5/1 -> AVR/5
  Constant6/1 -> AVR/6
  Constant7/1 -> AVR/7
  Constant8/1 -> AVR/8
  Constant9/1 -> AVR/9
  AVR/1 -> "E_FD Simulink-PS "/1
  Terminal Current PS-Simulink/1 -> AVR/4
  connections:
  "E_FD Simulink-PS "/RConn1 -- Exciter/LConn1
  I_FD PS-Simulink/LConn1 -- Exciter/LConn2
  fd-/RConn1 -- Exciter/RConn2
  Exciter/RConn1 -- fd+/RConn1
  Terminal Voltage Measurement/LConn1 -- Terminal Current Measurement/LConn1 -- pu/RConn1
  Terminal Voltage Measurement/RConn1 -- Terminal Voltage PS-Simulink/LConn1
  Terminal Current Measurement/RConn1 -- Terminal Current PS-Simulink/LConn1
